simulink model "vrtkoff_hud"  (Simulink 7.4)
settings: Solver=ode45  StartTime=0.0  StopTime=15  RelTol=1e-3
libraries: vrlib x3, aerospace x1
Description:
  | Plane Take-Off with HUD Text
  | 
  | This model is a variant of the vrtkoff example that shows also how to display
  | signal values as text in the virtual scene and a simple Head-Up Display (HUD).
  | 
  | The text is sent to virtual scene using the VR Text Output block. This block formats
  | the input vector using the format string defined in its mask (see sprintf() for more information)
  | and resulting string is sent to the 'string' field of the associated VRML text node in the scene.
  | 
  | The HUD behavior (maintaining constant relative position between the user and the
  | Text node) is achieved by defining a ProximitySensor that senses user position and
  | orientation as it navigates through the scene and routing this information to the translation
  | and rotation of HUD object - in this case a VRML Transform that contains the Text node.
settings Model: Creator=Straka  LastModifiedBy=Houska  CovMetricSettings=d  ExtModeTrigMode=oneshot  ExtModeArmWhenConnect=off
settings DataIOCC: SaveOutput=off  SaveTime=off  SignalLoggingName=logsOut
settings OptimizationCC: BlockReduction=off  BooleanDataType=off  InlineInvariantSignals=on  InitFltsAndDblsToZero=on
settings DebuggingCC: CheckExecutionContextPreStartOutputMsg=on  CheckExecutionContextRuntimeOutputMsg=on  SignalResolutionControl=TryResolveAllWithWarning  SolverPrmCheckMsg=none  MultiTaskDSMMsg=warning  MultiTaskCondExecSysMsg=none  StrictBusMsg=None
settings HardwareCC: TargetUnknown=on
settings ModelReferenceCC: UpdateModelReferenceTargets=IfOutOfDate
settings SFSimCC: SimGenerateEmlReport=off
settings RTWCC: IncludeERTFirstTime=on
settings GRTTargetCC: TargetFcnLib=ansi_tfl_tmw.mat

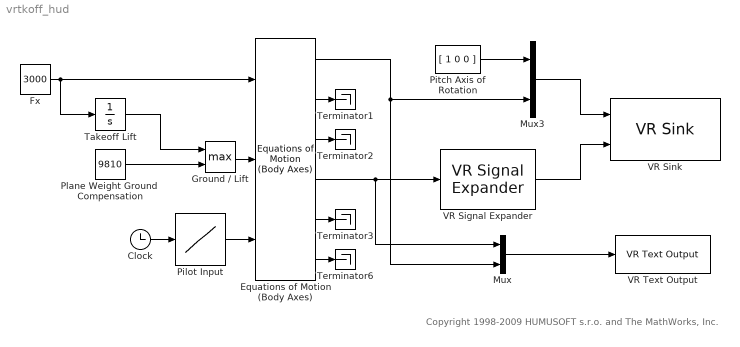
== system vrtkoff_hud ==
  note: Copyright 1998-2009 HUMUSOFT s.r.o. and The MathWorks, Inc.
  " Equations of Motion (Body Axes)" : aerospace/3DoF Equations of Motion / Equations of Motion (Body Axes)  SystemSampleTime=-1  v_ini=0  theta_ini=0  alpha_ini=0  q_ini=0  pos_ini=[0 0]  mass=1000  Iyy=1000  g=-9.81
  Clock : Clock
      settings: Decimation=10
  Fx : Constant  Value=3000  OutDataType=sfix(16)  OutScaling=2^0
  Ground / Lift : MinMax  Function=max  Inputs=2  OutDataType=sfix(16)  OutScaling=2^0  ZeroCross=off  SaturateOnIntegerOverflow=on  InputSameDT=on
  Mux : Mux  Inputs=2
  Mux3 : Mux  Inputs=2
  Pilot Input : Lookup  InputValues=[0 1 2 8 9 15]  Table=[0 0 -20 20 0 0]  OutDataType=sfix(16)  OutScaling=2^0  SaturateOnIntegerOverflow=on
  Pitch Axis of Rotation : Constant  Value=[ 1 0 0 ]  OutDataType=sfix(16)  OutScaling=2^0
  Plane Weight Ground  Compensation : Constant  Value=9810  OutDataType=sfix(16)  OutScaling=2^0
  Takeoff Lift : Integrator  LimitOutput=on  UpperSaturationLimit=11000  LowerSaturationLimit=-Inf  ZeroCross=off
  Terminator{1..3,6} (4 alike) : Terminator
  VR Signal Expander : vrlib/VR Signal Expander  SystemSampleTime=-1  outwidth=3  outidx=[3 2]
  VR Sink : vrlib/VR Sink  InstantiateOnLoad=on  SampleTime=0.05  ViewEnable=on  RemoteChange=off  RemoteView=off  FieldsWritten=Plane.rotation.4.1.double#Plane.translation.3.1.double  WorldFileName=vrtkoff_hud.wrl  WorldDescription=VR Plane Take-Off with HUD Text  AutoView=on  VideoDimensions=[]  FigureProperties="{'Position', 'Name', 'Viewpoint', 'CameraBound', 'CameraDirection', 'CameraPosition', 'CameraUpVector', 'ZoomFactor', 'Antialiasing', 'Headlight', 'Lighting', 'NavPanel', 'StatusBar', 'ToolBar', 'Textures', 'Transparency', 'Wireframe', 'NavZones', 'NavMode', 'NavSpeed', 'Record2DCompressMethod', 'Record2DCompressQuality', 'Record2D', 'Record2DFileName', 'Record2DFPS'; [1.5000000000000000e+001  7.8000000000000000e+001  5.7600000000000000e+002  3.8000000000000000e+002], 'VR Plane Take-Off with HUD Text', 'Airport', 'on', [0.0000000000000000e+000  0.0000000000000000e+000 -1.0000000000000000e+000], [0.0000000000000000e+000  0.0000000000000000e+000  0.0000000000000000e+000], [0.0000000000000000e+000  1.0000000000000000e+000  0.0000000000000000e+000], [1.0000000000000000e+000], 'off', 'on', 'on', 'halfbar', 'on', 'on', 'on', 'on', 'off', 'off', 'fly', 'normal', 'auto', [7.5000000000000000e+001], 'off', '%f_anim_%n.avi', [1.5000000000000000e+001]}"
  VR Text Output : vrlib/VR Text Output  VrmlFile=vrtkoff_hud.wrl  TxtNode=HUDText1  FormatString="Xe      : %7.2f m\\nZe      : %7.2f m\\nAttitude: %7.2f rad"  Ts=0.05  ForceViewerOpen=off
  wires:
  Pitch Axis of Rotation/1 -> Mux3/1
  Mux3/1 -> VR Sink/1
  VR Signal Expander/1 -> VR Sink/2
  " Equations of Motion (Body Axes)"/2 -> Terminator1/1
  " Equations of Motion (Body Axes)"/3 -> Terminator2/1
  Ground / Lift/1 -> " Equations of Motion (Body Axes)"/2
  Takeoff Lift/1 -> Ground / Lift/1
  Plane Weight Ground  Compensation/1 -> Ground / Lift/2
  Clock/1 -> Pilot Input/1
  Pilot Input/1 -> " Equations of Motion (Body Axes)"/3
  Fx/1 -> " Equations of Motion (Body Axes)"/1, Takeoff Lift/1
  " Equations of Motion (Body Axes)"/6 -> Terminator6/1
  " Equations of Motion (Body Axes)"/5 -> Terminator3/1
  " Equations of Motion (Body Axes)"/1 -> Mux3/2, Mux/2
  " Equations of Motion (Body Axes)"/4 -> VR Signal Expander/1, Mux/1
  Mux/1 -> VR Text Output/1
